simulink model "Example_2_1"  (R2018a)
settings: Solver=VariableStepAuto  StartTime=0.0  StopTime=Tsim  RelTol=1e-3
InitFcn:
  | parameters
values from neighbouring files (symbols this model uses):
  A = [0 0 ... (first row only)    [parameters.m]
  B = [1 ... (first row only)    [parameters.m]
  F = [-4*exp(h)+1  -4*exp(h)]    [parameters.m]
  h = 1    [parameters.m]
  s = tf('s')    [parameters.m]
undefined symbols (not defined in the file or in its folder): BA
libraries: cstblocks x3
settings Model: PauseTimes=5.5  Creator=adriano  LastModifiedBy=controle

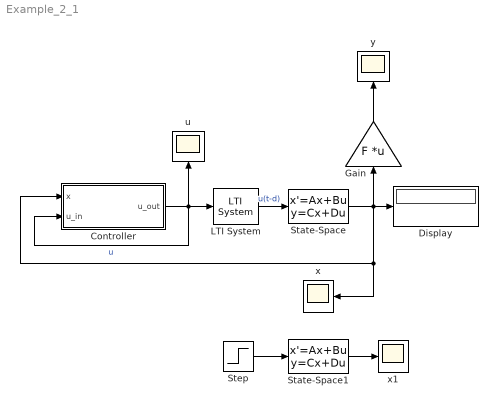
== system Example_2_1 ==
  Controller : Subsystem
  Display : Display
  Gain : Gain  Gain=F  Multiplication=Matrix(K*u)
  LTI System : cstblocks/LTI System  sys=exp(-s*h)  IC=[]
  State-Space : StateSpace  A=A  B=BA  C=eye(2)  D=zeros(2,1)  InitialCondition=[.1 0]
  State-Space1 : StateSpace  A=A  B=B  C=eye(2)  D=zeros(2,1)  InitialCondition=[.1 0]
  Step : Step  SampleTime=0
  u : Scope
  x : Scope
  x1 : Scope
  y : Scope
  wires:
  Controller/1(u_out) -> LTI System/1, u/1, Controller/2(u_in)  "u"
  LTI System/1 -> State-Space/1  "u(t-d)"
  Gain/1 -> y/1
  State-Space/1 -> x/1, Controller/1(x), Display/1, Gain/1
  Step/1 -> State-Space1/1
  State-Space1/1 -> x1/1

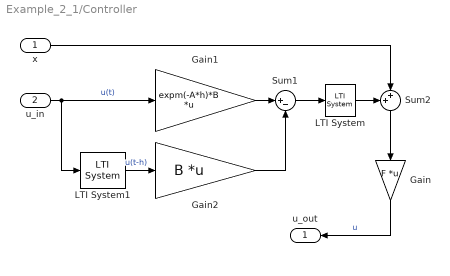
== system Example_2_1/Controller ==
  x : Inport
  u_in : Inport  Port=2
  Gain : Gain  Gain=F  Multiplication=Matrix(K*u)
  Gain1 : Gain  Gain=expm(-A*h)*B  Multiplication=Matrix(K*u)
  Gain2 : Gain  Gain=B  Multiplication=Matrix(K*u)
  LTI System : cstblocks/LTI System  sys=S  IC=[]
  LTI System1 : cstblocks/LTI System  sys=exp(-s*h)  IC=[]
  Sum1 : Sum  Inputs=|+-
  Sum2 : Sum  Inputs=++|
  u_out : Outport
  wires:
  Sum2/1 -> Gain/1
  u_in/1 -> LTI System1/1, Gain1/1  "u(t)"
  LTI System1/1 -> Gain2/1  "u(t-h)"
  Gain1/1 -> Sum1/1
  Gain2/1 -> Sum1/2
  Sum1/1 -> LTI System/1
  LTI System/1 -> Sum2/1
  x/1 -> Sum2/2
  Gain/1 -> u_out/1  "u"
